simulink model "laserSim"  (R2022b)
settings: Solver=VariableStepAuto  StartTime=0.0  StopTime=t  RelTol=1e-3
values from neighbouring files (symbols this model uses):
  dutyCycle = power/100    (= 0.1)    [simulationLIGFabricatedScript.m]
  F = 80000    [simulationLIGFabricatedScript.m]
  powerMax = 25    [simulationLIGFabricatedScript.m]
  tau = 40e-6    (= 4e-05)    [simulationLIGFabricatedScript.m]
libraries: simulink x1
settings Model: Creator=MinosPortatil2  LastModifiedBy=MinosPortatil2

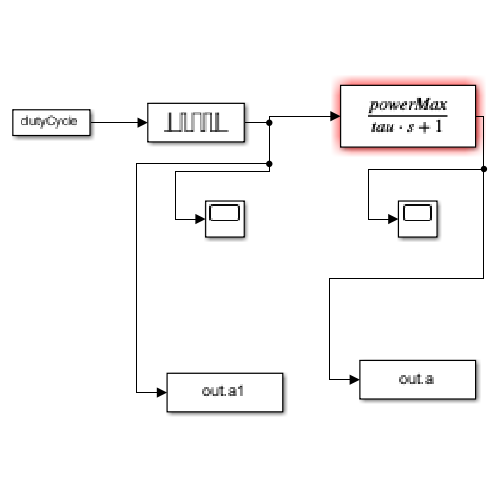
[thumbnail: Simulink's stored preview of the top-level diagram]
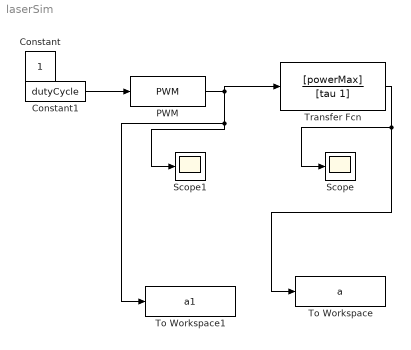
== system laserSim ==
  Constant1 : Constant  Value=dutyCycle
  PWM : simulink/Discontinuities/PWM  DisableCoverage=on  Period=1/F  InitialDelay=0  DisallowZeroDutyCycle=off  RunAtFixedTimeIntervals=off  SampleTime=1/(6*F)
  Scope : Scope
  Scope1 : Scope
  To Workspace : ToWorkspace  VariableName=a  SampleTime=-1
  To Workspace1 : ToWorkspace  VariableName=a1  SampleTime=-1
  Transfer Fcn : TransferFcn  Numerator=[powerMax]  Denominator=[tau 1]
  Constant : Constant  IOType=siggen
  wires:
  Constant1/1 -> PWM/1
  PWM/1 -> To Workspace1/1, Scope1/1, Transfer Fcn/1
  Transfer Fcn/1 -> Scope/1, To Workspace/1
